simulink model "robopd"  (Simulink 7.7)
settings: Solver=ode45  StartTime=0.0  StopTime=50  MaxStep=0.1  RelTol=1e-4
undefined symbols (not defined in the file or in its folder): q0
settings Model: Creator=fernando  LastModifiedBy=fernando  ExtModeAutoUpdateStatusClock=off
settings OptimizationCC: InitFltsAndDblsToZero=on
settings DebuggingCC: SaveWithParameterizedLinksMsg=none  SignalResolutionControl=TryResolveAllWithWarning  MultiTaskDSMMsg=warning  MultiTaskCondExecSysMsg=none  StrictBusMsg=None
settings SFSimCC: SimParseCustomCode=off
settings RTWCC: IncludeERTFirstTime=on
settings GRTTargetCC: TargetFcnLib=ansi_tfl_tmw.mat

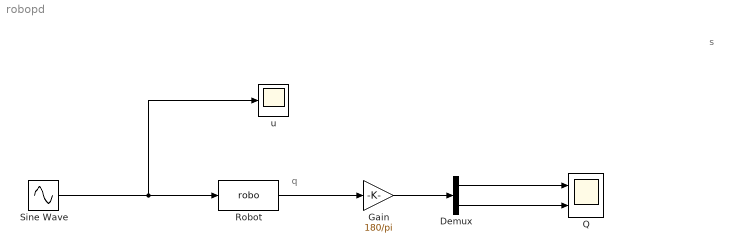
== system robopd ==
  note: q
  note: s
  Demux : Demux  Outputs=2
  Gain : Gain  Gain=180/pi
  Q : Scope  NumInputPorts=2
      settings: YMin=-1.75~-0.05  YMax=3.25~0.7
  Robot : S-Function  FunctionName=robo  Parameters=q0  EnableBusSupport=off  mask(Robot){xi=q0}
      mask prompts: xi "Condicao Inicial"
  Sine Wave : Sin  Amplitude=[1;1]*1000  Frequency=[1;0.5]  SampleTime=0
  u : Scope
      settings: YMin=-0.175  YMax=0.225  SaveName=ScopeData6
  wires:
  Robot/1 -> Gain/1
  Demux/2 -> Q/2
  Demux/1 -> Q/1
  Sine Wave/1 -> Robot/1, u/1
  Gain/1 -> Demux/1
